simulink model "Schnittstellendummy_Gewerk3"  (R2015b)
settings: Solver=VariableStepAuto  StartTime=0.0  StopTime=100.0  RelTol=1e-3
settings Model: Creator=atlabor  LastModifiedBy=atlabor

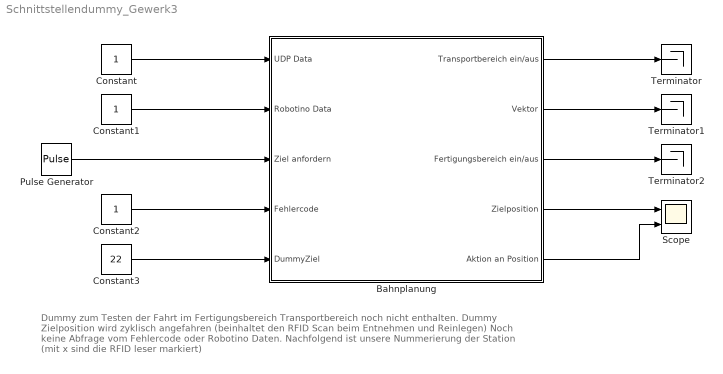
== system Schnittstellendummy_Gewerk3 ==
  note: Dummy zum Testen der Fahrt im Fertigungsbereich Transportbereich noch nicht enthalten.
      | Dummy Zielposition wird zyklisch angefahren (beinhaltet den RFID Scan beim Entnehmen und Reinlegen)
      | Noch keine Abfrage vom Fehlercode oder Robotino Daten.
      | Nachfolgend ist unsere Nummerierung der Station (mit x sind die RFID leser markiert)
  Bahnplanung : Subsystem
  Constant : Constant
  Constant1 : Constant
  Constant2 : Constant
  Constant3 : Constant  Value=22
  Pulse Generator : DiscretePulseGenerator  PulseType=Time based  Period=5  PulseWidth=50
  Scope : Scope  NumInputPorts=2
  Terminator : Terminator
  Terminator1 : Terminator
  Terminator2 : Terminator
  wires:
  Constant/1 -> Bahnplanung/1(UDP Data)
  Constant1/1 -> Bahnplanung/2("Robotino Data ")
  Constant2/1 -> Bahnplanung/4(Fehlercode)
  Constant3/1 -> Bahnplanung/5(DummyZiel)
  Bahnplanung/1(Transportbereich ein/aus) -> Terminator/1
  Bahnplanung/2(Vektor) -> Terminator1/1
  Bahnplanung/3(Fertigungsbereich ein/aus) -> Terminator2/1
  Bahnplanung/4(Zielposition) -> Scope/1
  Bahnplanung/5(Aktion an Position) -> Scope/2
  Pulse Generator/1 -> Bahnplanung/3(Ziel anfordern)

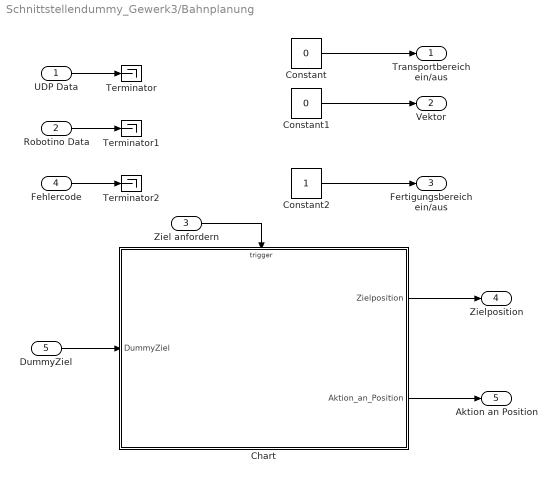
== system Schnittstellendummy_Gewerk3/Bahnplanung ==
  UDP Data : Inport
  "Robotino Data " : Inport  Port=2
  Ziel anfordern : Inport  Port=3
  Fehlercode : Inport  Port=4
  DummyZiel : Inport  Port=5
  Chart : Stateflow chart  TreatAsAtomicUnit=on
  Constant : Constant  Value=0
  Constant1 : Constant  Value=0
  Constant2 : Constant
  Terminator : Terminator
  Terminator1 : Terminator
  Terminator2 : Terminator
  Transportbereich ein/aus : Outport
  Vektor : Outport  Port=2
  Fertigungsbereich ein/aus : Outport  Port=3
  Zielposition : Outport  Port=4
  Aktion an Position : Outport  Port=5
  wires:
  Constant1/1 -> Vektor/1
  Constant/1 -> Transportbereich ein/aus/1
  Constant2/1 -> Fertigungsbereich ein/aus/1
  UDP Data/1 -> Terminator/1
  "Robotino Data "/1 -> Terminator1/1
  Fehlercode/1 -> Terminator2/1
  Chart/1(Zielposition) -> Zielposition/1
  Chart/2(Aktion_an_Position) -> Aktion an Position/1
  Ziel anfordern/1 -> Chart/Trigger
  DummyZiel/1 -> Chart/1(DummyZiel)

== stateflow chart Schnittstellendummy_Gewerk3/Bahnplanung/Chart ==
  settings: sampleTime=0.01
  state Fertigungsbereich
    entry:Werkstueck=0;
    state RFID_einchecken
      entry:Zielposition=DummyZiel-mod(DummyZiel,10)+3,
      Aktion_an_Position=Aktion_Warten;
    state Startpunkt
      entry: Zielposition=DummyZiel-mod(DummyZiel,10);
      Aktion_an_Position=Aktion_Warten;
    state Warten
    state Position_anfahren
      entry:Zielposition=DummyZiel,
      if(Werkstueck==0) Aktion_an_Position=Aktion_Aufnehmen,
      Werkstueck=1;
      else Aktion_an_Position=Aktion_Ablegen,
      Werkstueck=0;
      end
    state Bereich_verlassen
      entry:Zielposition=DummyZiel-mod(DummyZiel,10)+4,
      Aktion_an_Position=Aktion_Warten;
    state RFID_auschecken
      entry:Zielposition=DummyZiel-mod(DummyZiel,10)+3,
      Aktion_an_Position=Aktion_Warten;
    Startpunkt -> RFID_einchecken [order 1] : [Ziel_anfordern & Werkstueck==1]
    (default) -> Startpunkt
    Startpunkt -> Position_anfahren [order 2] : [Ziel_anfordern & Werkstueck==0]
    Warten -> Startpunkt : after(Wartezeit,sec)
    RFID_einchecken -> Position_anfahren : after(Wartezeit,sec)
    Bereich_verlassen -> Warten : Ziel_anfordern
    Position_anfahren -> Bereich_verlassen [order 2] : [Ziel_anfordern & Werkstueck==0]
    Position_anfahren -> RFID_auschecken [order 1] : [Ziel_anfordern & Werkstueck==1]
    RFID_auschecken -> Bereich_verlassen : after(Wartezeit,sec)
  data: DummyZiel input; Zielposition output; Aktion_an_Position output; Aktion_Warten local double =2; Aktion_Aufnehmen local double =1; Aktion_Ablegen local double =0; Werkstueck local double; Wartezeit local double =5
  events: Ziel_anfordern input RISING_EDGE_EVENT
